simulink model "px4_mc_notch_sim"  (R2019b)
settings: Solver=FixedStepAuto  StartTime=0.0  StopTime=sim_time  FixedStep=1/sim_freq  RelTol=1e-3
values from neighbouring files (symbols this model uses):
  notch = (s^2 + wc^2)/(s^2 + o*s + wc^2)    [notch_design.m]
  pos_e_step = [0,2,0]    [run_sim.m]
  pulse_amplitude = 0.1    [run_sim.m]
  pulse_period = 40    [run_sim.m]
  ramp_max = 0.5    [run_sim.m]
  ramp_slope = 0.05    [run_sim.m]
  sinus_amplitude = 0.1    [run_sim.m]
  sinus_bias = 0    [run_sim.m]
  sinus_freq = 5    [run_sim.m]
  step_delay = 1    [run_sim.m]
  step_mag = 0.5    [run_sim.m]
  yaw_step = 0.00    (= 0)    [run_sim.m]
undefined symbols (not defined in the file or in its folder): br_filt_denom, br_filt_num, C_D, d, DiscIntNeverNeededParam, eta_w, g, hover_perc, m, max_T, MC_PITCH_P, MC_PITCHRATE_D, MC_PITCHRATE_I, MC_PITCHRATE_MAX, MC_PITCHRATE_P, MC_PR_INT_LIM, MC_ROLL_P, MC_ROLLRATE_D, MC_ROLLRATE_I, MC_ROLLRATE_MAX, MC_ROLLRATE_P, MC_RR_INT_LIM, MC_YAW_P, MC_YAWRATE_D, MC_YAWRATE_I, MC_YAWRATE_MAX, MC_YAWRATE_P, MC_YR_INT_LIM, MPC_THR_MAX, MPC_THR_MIN, MPC_TILTMAX_AIR, MPC_XY_P, MPC_XY_VEL_D, MPC_XY_VEL_I, MPC_XY_VEL_MAX, MPC_XY_VEL_P, MPC_Z_P, MPC_Z_VEL_D, MPC_Z_VEL_I, MPC_Z_VEL_MAX_DN, MPC_Z_VEL_MAX_UP, MPC_Z_VEL_P, r_D, rho, tau_T, vel_filt_denom, vel_filt_num, virtual_controls_mat, wind
libraries: simulink x7, sharedtransform x2, shared6dof x1
settings Model: Creator=henry  LastModifiedBy=henry

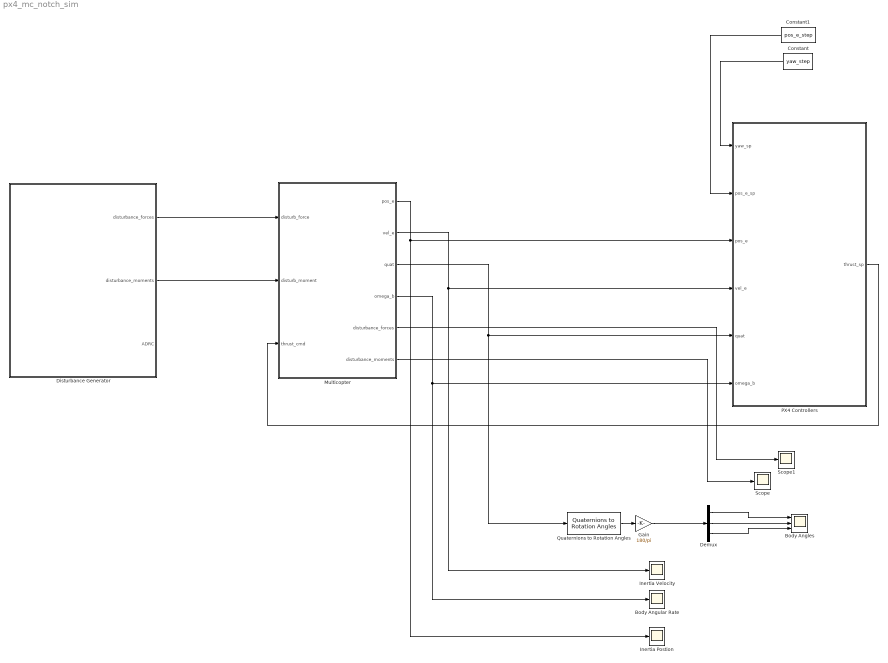
== system px4_mc_notch_sim ==
  Body Angles : Scope  NumInputPorts=3
  Body Angular Rate : Scope
  Constant : Constant  Value=yaw_step
  Constant1 : Constant  Value=pos_e_step
  Demux : Demux  Outputs=3
  Disturbance Generator : Subsystem
  Gain : Gain  Gain=180/pi
  Inertia Postion : Scope
  Inertia Velocity : Scope
  Multicopter : Subsystem
  PX4 Controllers : Subsystem
  Quaternions to Rotation Angles : sharedtransform/Quaternions to Rotation Angles  rotationOrder=XYZ  aMode=aMode
      settings: SourceProductBaseCode=AE
  Scope : Scope
  Scope1 : Scope
  wires:
  Multicopter/4(omega_b) -> Body Angular Rate/1, PX4 Controllers/6(omega_b)
  Multicopter/3("quat ") -> PX4 Controllers/5(quat), Quaternions to Rotation Angles/1
  Multicopter/1(pos_e) -> Inertia Postion/1, PX4 Controllers/3(pos_e)
  Multicopter/2(vel_e) -> PX4 Controllers/4(vel_e), Inertia Velocity/1
  PX4 Controllers/1(thrust_sp) -> Multicopter/3(thrust_cmd)
  Constant/1 -> PX4 Controllers/1(yaw_sp)
  Constant1/1 -> PX4 Controllers/2(pos_e_sp)
  Quaternions to Rotation Angles/1 -> Gain/1
  Multicopter/5(disturbance_forces) -> Scope1/1
  Gain/1 -> Demux/1
  Demux/1 -> Body Angles/1
  Demux/2 -> Body Angles/2
  Demux/3 -> Body Angles/3
  Disturbance Generator/2(disturbance_moments) -> Multicopter/2(disturb_moment)
  Disturbance Generator/1(disturbance_forces) -> Multicopter/1(disturb_force)
  Multicopter/6(disturbance_moments) -> Scope/1

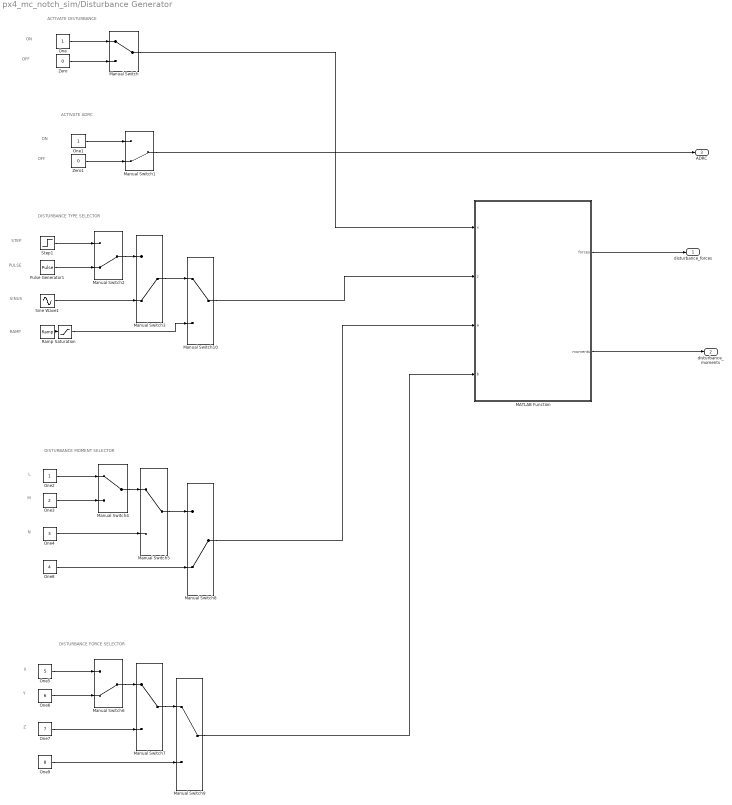
== system px4_mc_notch_sim/Disturbance Generator ==
  note: STEP
  note: OFF
  note: ON
  note: ACTIVATE DISTURBANCE
  note: DISTURBANCE TYPE SELECTOR
  note: ACTIVATE ADRC
  note: OFF
  note: ON
  note: PULSE
  note: SINUS
  note: N
  note: DISTURBANCE MOMENT SELECTOR
  note: M
  note: L
  note: Z
  note: X
  note: Y
  note: DISTURBANCE FORCE SELECTOR
  note: RAMP
  MATLAB Function : MATLAB Function  TreatAsAtomicUnit=on
  Manual Switch{,4..5,7,9..10} (6 alike) : ManualSwitch
  Manual Switch{1..3,6,8} (5 alike) : ManualSwitch  CurrentSetting=0
  One : Constant  OutDataTypeStr=Inherit: Inherit via back propagation
  One1 : Constant  OutDataTypeStr=Inherit: Inherit via back propagation
  One2 : Constant  OutDataTypeStr=Inherit: Inherit via back propagation
  One3 : Constant  Value=2  OutDataTypeStr=Inherit: Inherit via back propagation
  One4 : Constant  Value=3  OutDataTypeStr=Inherit: Inherit via back propagation
  One5 : Constant  Value=5  OutDataTypeStr=Inherit: Inherit via back propagation
  One6 : Constant  Value=6  OutDataTypeStr=Inherit: Inherit via back propagation
  One7 : Constant  Value=7  OutDataTypeStr=Inherit: Inherit via back propagation
  One8 : Constant  Value=4  OutDataTypeStr=Inherit: Inherit via back propagation
  One9 : Constant  Value=8  OutDataTypeStr=Inherit: Inherit via back propagation
  Pulse Generator1 : DiscretePulseGenerator  PulseType=Time based  Amplitude=pulse_amplitude  Period=pulse_period  PulseWidth=50
  Ramp : simulink/Sources/Ramp  slope=ramp_slope  start=ramp_start  InitialOutput=0
  Saturation : Saturate  UpperLimit=ramp_max  LowerLimit=0
  Sine Wave1 : Sin  Amplitude=sinus_amplitude  Bias=sinus_bias  Frequency=sinus_freq  SampleTime=0
  Step1 : Step  Time=step_delay  After=step_mag  SampleTime=0
  Zero : Constant  Value=0  OutDataTypeStr=Inherit: Inherit via back propagation
  Zero1 : Constant  Value=0  OutDataTypeStr=Inherit: Inherit via back propagation
  disturbance_forces : Outport
  disturbance_moments : Outport  Port=2
  ADRC : Outport  Port=3
  wires:
  One6/1 -> Manual Switch6/2
  Manual Switch7/1 -> Manual Switch9/1
  One8/1 -> Manual Switch8/2
  One7/1 -> Manual Switch7/2
  Manual Switch5/1 -> Manual Switch8/1
  One9/1 -> Manual Switch9/2
  One3/1 -> Manual Switch4/2
  Manual Switch6/1 -> Manual Switch7/1
  One5/1 -> Manual Switch6/1
  Pulse Generator1/1 -> Manual Switch2/2
  Sine Wave1/1 -> Manual Switch3/2
  Manual Switch4/1 -> Manual Switch5/1
  Manual Switch8/1 -> MATLAB Function/3(a)
  One/1 -> Manual Switch/1
  MATLAB Function/1(forces) -> disturbance_forces/1
  Zero/1 -> Manual Switch/2
  Manual Switch9/1 -> MATLAB Function/4(b)
  Zero1/1 -> Manual Switch1/2
  One4/1 -> Manual Switch5/2
  Manual Switch/1 -> MATLAB Function/1(x)
  MATLAB Function/2(moments) -> disturbance_moments/1
  Manual Switch2/1 -> Manual Switch3/1
  Step1/1 -> Manual Switch2/1
  One1/1 -> Manual Switch1/1
  One2/1 -> Manual Switch4/1
  Manual Switch1/1 -> ADRC/1
  Ramp/1 -> Saturation/1
  Manual Switch3/1 -> Manual Switch10/1
  Saturation/1 -> Manual Switch10/2
  Manual Switch10/1 -> MATLAB Function/2(z)

== system px4_mc_notch_sim/Multicopter ==
  disturb_force : Inport
  disturb_moment : Inport  Port=2
  thrust_cmd : Inport  Port=3
  6 DOF MODEL : Subsystem
  Forces and Moments : Subsystem
  Motor Model : Subsystem
  pos_e : Outport
  vel_e : Outport  Port=2
  "quat " : Outport  Port=3
  omega_b : Outport  Port=4
  disturbance_forces : Outport  Port=5
  disturbance_moments : Outport  Port=6
  wires:
  6 DOF MODEL/1(vel_b) -> Forces and Moments/1(vel_b)
  6 DOF MODEL/3(qaut) -> Forces and Moments/3(quat), "quat "/1
  6 DOF MODEL/2(pos_e) -> pos_e/1, Forces and Moments/2(pos_e)
  Forces and Moments/2(moments) -> 6 DOF MODEL/2(moments)
  6 DOF MODEL/5(omega_b) -> omega_b/1
  6 DOF MODEL/4(vel_e) -> vel_e/1
  Forces and Moments/1(forces) -> 6 DOF MODEL/1("forces ")
  thrust_cmd/1 -> Motor Model/1(thrust_cmd)
  Motor Model/1(force) -> Forces and Moments/4(thrust_cmd)
  Forces and Moments/3(disturbance_force) -> disturbance_forces/1
  Forces and Moments/4(disturbance_moments) -> disturbance_moments/1
  disturb_force/1 -> Forces and Moments/5(disturb_force)
  disturb_moment/1 -> Forces and Moments/6(disturb_moments)

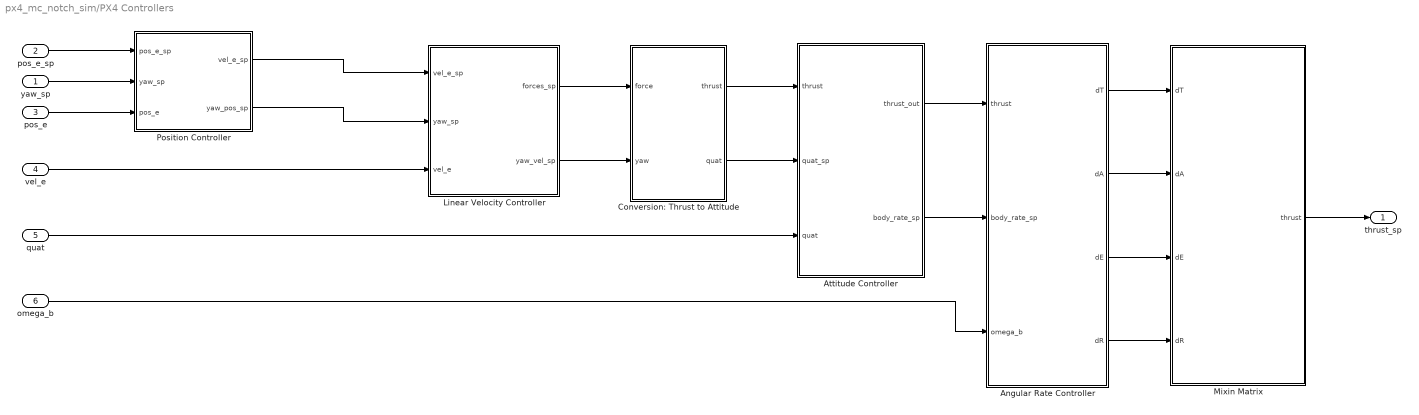
== system px4_mc_notch_sim/PX4 Controllers ==
  yaw_sp : Inport
  pos_e_sp : Inport  Port=2
  pos_e : Inport  Port=3
  vel_e : Inport  Port=4
  quat : Inport  Port=5
  omega_b : Inport  Port=6
  Angular Rate Controller : Subsystem
  Attitude Controller : Subsystem
  Conversion: Thrust to Attitude : Subsystem
  Linear Velocity Controller : Subsystem
  Mixin Matrix : Subsystem
  Position Controller : Subsystem
  thrust_sp : Outport
  wires:
  yaw_sp/1 -> Position Controller/2(yaw_sp)
  pos_e_sp/1 -> Position Controller/1(pos_e_sp)
  quat/1 -> Attitude Controller/3(quat)
  omega_b/1 -> Angular Rate Controller/3(omega_b)
  pos_e/1 -> Position Controller/3(pos_e)
  vel_e/1 -> Linear Velocity Controller/3(vel_e)
  Position Controller/2(yaw_pos_sp) -> Linear Velocity Controller/2(yaw_sp)
  Position Controller/1(vel_e_sp) -> Linear Velocity Controller/1(vel_e_sp)
  Linear Velocity Controller/1(forces_sp) -> Conversion: Thrust to Attitude/1(force)
  Linear Velocity Controller/2(yaw_vel_sp) -> Conversion: Thrust to Attitude/2(yaw)
  Conversion: Thrust to Attitude/1(thrust) -> Attitude Controller/1(thrust)
  Conversion: Thrust to Attitude/2(quat) -> Attitude Controller/2(quat_sp)
  Attitude Controller/1(thrust_out) -> Angular Rate Controller/1(thrust)
  Attitude Controller/2(body_rate_sp) -> Angular Rate Controller/2(body_rate_sp)
  Angular Rate Controller/1(dT) -> Mixin Matrix/1(dT)
  Angular Rate Controller/2(dA) -> Mixin Matrix/2(dA)
  Angular Rate Controller/3(dE) -> Mixin Matrix/3(dE)
  Angular Rate Controller/4(dR) -> Mixin Matrix/4(dR)
  Mixin Matrix/1(thrust) -> thrust_sp/1

== system px4_mc_notch_sim/Multicopter/6 DOF MODEL ==
  "forces " : Inport
  moments : Inport  Port=2
  6DOF (Quaternion) : shared6dof/6DOF (Euler Angles)  units=Metric (MKS)  mtype=Fixed  rep=Quaternion  xme_0=[0 0 0]  Vm_0=[0 0 0]  eul_0=[0 0 0]  pm_0=[0 0 0]  mass_0=m  mass_e=0.5  mass_f=2.0  inertia=I  inertia_e=eye(3)  inertia_f=2*eye(3)  k_quat=2  vre_flag=on  abi_flag=off  aMode=0  xme_statename=''  Vm_statename=''  eul_statename=''  quat_statename=''  pm_statename=''  mass_statename=''
      settings: SourceProductBaseCode=AE
  Direction Cosine Matrix to Quaternions : sharedtransform/Direction Cosine Matrix  to Quaternions  aMode=0  action=None  tolerance=eps(2)
      settings: SourceProductName=Aerospace Blockset  SourceProductBaseCode=AE
  Terminator : Terminator
  Terminator1 : Terminator
  Terminator2 : Terminator
  vel_b : Outport
  pos_e : Outport  Port=2
  qaut : Outport  Port=3
  vel_e : Outport  Port=4
  omega_b : Outport  Port=5
  wires:
  "forces "/1 -> 6DOF (Quaternion)/1
  moments/1 -> 6DOF (Quaternion)/2
  6DOF (Quaternion)/8 -> Terminator/1
  6DOF (Quaternion)/7 -> Terminator1/1
  6DOF (Quaternion)/3 -> Terminator2/1
  6DOF (Quaternion)/1 -> vel_e/1
  6DOF (Quaternion)/2 -> pos_e/1
  6DOF (Quaternion)/5 -> vel_b/1
  6DOF (Quaternion)/6 -> omega_b/1
  Direction Cosine Matrix to Quaternions/1 -> qaut/1
  6DOF (Quaternion)/4 -> Direction Cosine Matrix to Quaternions/1

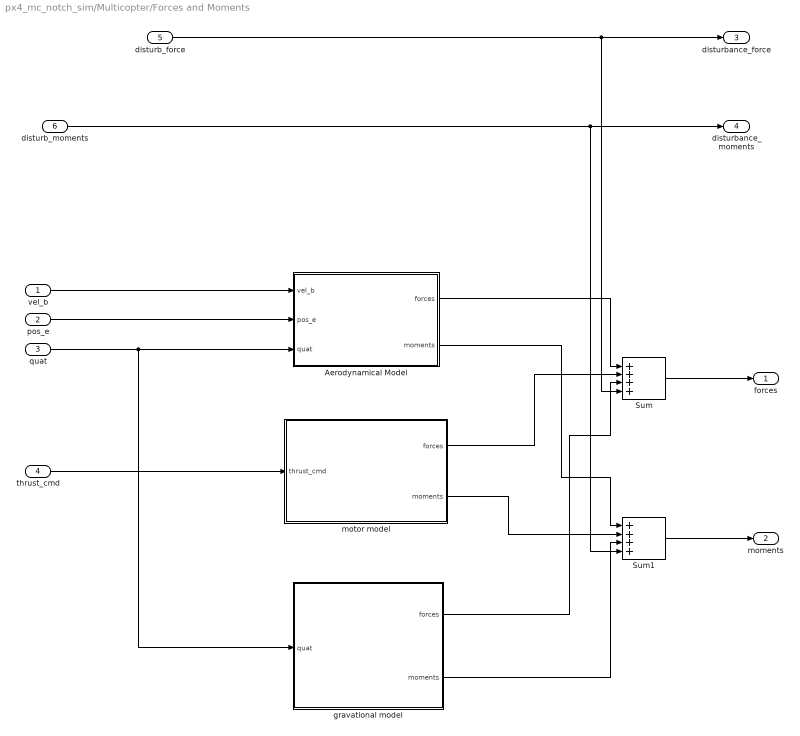
== system px4_mc_notch_sim/Multicopter/Forces and Moments ==
  vel_b : Inport
  pos_e : Inport  Port=2
  quat : Inport  Port=3
  thrust_cmd : Inport  Port=4
  disturb_force : Inport  Port=5
  disturb_moments : Inport  Port=6
  Aerodynamical Model : Subsystem
  Sum : Sum  Inputs=++++
  Sum1 : Sum  Inputs=++++
  gravational model : Subsystem
  motor model : Subsystem
  forces : Outport
  moments : Outport  Port=2
  disturbance_force : Outport  Port=3
  disturbance_moments : Outport  Port=4
  wires:
  Sum/1 -> forces/1
  Sum1/1 -> moments/1
  motor model/1(forces) -> Sum/2
  motor model/2(moments) -> Sum1/2
  gravational model/1(forces) -> Sum/3
  gravational model/2(moments) -> Sum1/3
  vel_b/1 -> Aerodynamical Model/1(vel_b)
  pos_e/1 -> Aerodynamical Model/2(pos_e)
  Aerodynamical Model/1(forces) -> Sum/1
  Aerodynamical Model/2(moments) -> Sum1/1
  thrust_cmd/1 -> motor model/1(thrust_cmd)
  disturb_moments/1 -> Sum1/4, disturbance_moments/1
  quat/1 -> Aerodynamical Model/3(quat), gravational model/1(quat)
  disturb_force/1 -> Sum/4, disturbance_force/1

== system px4_mc_notch_sim/Multicopter/Motor Model ==
  thrust_cmd : Inport
  Linear Gain : Gain  Gain=max_T
  force : Outport  VectorParamsAs1DForOutWhenUnconnected=off
  wires:
  thrust_cmd/1 -> Linear Gain/1
  Linear Gain/1 -> force/1

== system px4_mc_notch_sim/PX4 Controllers/Angular Rate Controller ==
  thrust : Inport
  body_rate_sp : Inport  Port=2
  omega_b : Inport  Port=3
  Demux : Demux  Outputs=3
  Demux1 : Demux  Outputs=3
  Pitch Rate Controller : Subsystem
  Roll Rate Controller : Subsystem
  Yaw Rate Controller : Subsystem
  dT : Outport  VectorParamsAs1DForOutWhenUnconnected=off
  dA : Outport  Port=2  VectorParamsAs1DForOutWhenUnconnected=off
  dE : Outport  Port=3  VectorParamsAs1DForOutWhenUnconnected=off
  dR : Outport  Port=4  VectorParamsAs1DForOutWhenUnconnected=off
  wires:
  Demux1/3 -> Yaw Rate Controller/2(r)
  Demux/3 -> Yaw Rate Controller/1(rref)
  Demux1/1 -> Roll Rate Controller/2(p)
  thrust/1 -> dT/1
  Yaw Rate Controller/1(dR) -> dR/1
  Pitch Rate Controller/1(dE) -> dE/1
  Demux1/2 -> Pitch Rate Controller/2(q)
  Roll Rate Controller/1(dA) -> dA/1
  Demux/1 -> Roll Rate Controller/1(pref)
  Demux/2 -> Pitch Rate Controller/1(qref)
  omega_b/1 -> Demux1/1
  body_rate_sp/1 -> Demux/1

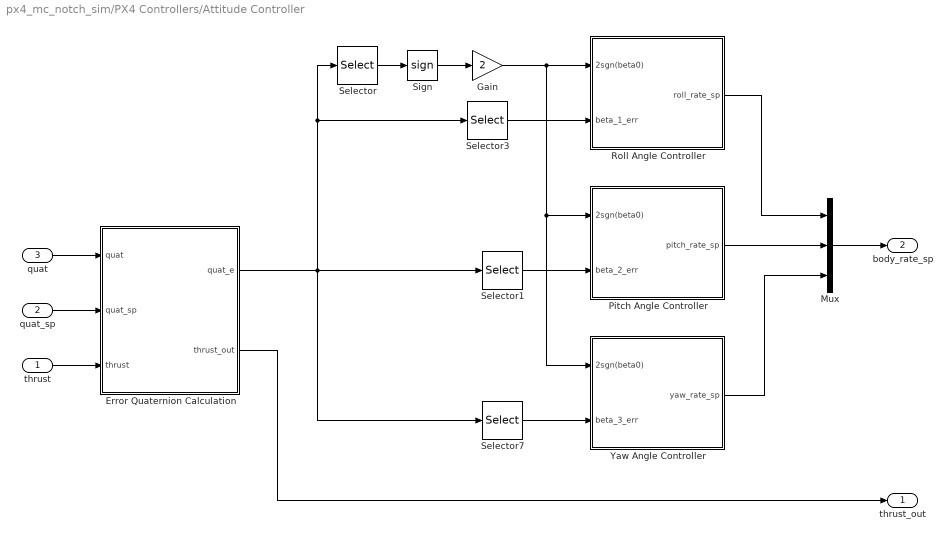
== system px4_mc_notch_sim/PX4 Controllers/Attitude Controller ==
  thrust : Inport  PortDimensions=1
  quat_sp : Inport  Port=2  PortDimensions=4
  quat : Inport  Port=3  PortDimensions=4
  Error Quaternion Calculation : MATLAB Function  TreatAsAtomicUnit=on
  Gain : Gain  Gain=2
  Mux : Mux  Inputs=3
  Pitch Angle Controller : Subsystem
  Roll Angle Controller : Subsystem
  Selector : Selector  InputPortWidth=4  IndexOptions=Index vector (dialog)  Indices=1  OutputSizes=1
  Selector1 : Selector  InputPortWidth=4  IndexOptions=Index vector (dialog)  Indices=3  OutputSizes=1
  Selector3 : Selector  InputPortWidth=4  IndexOptions=Index vector (dialog)  Indices=2  OutputSizes=1
  Selector7 : Selector  InputPortWidth=4  IndexOptions=Index vector (dialog)  Indices=4  OutputSizes=1
  Sign : Signum
  Yaw Angle Controller : Subsystem
  thrust_out : Outport  VectorParamsAs1DForOutWhenUnconnected=off
  body_rate_sp : Outport  Port=2  VectorParamsAs1DForOutWhenUnconnected=off
  wires:
  Pitch Angle Controller/1(pitch_rate_sp) -> Mux/2
  Selector7/1 -> Yaw Angle Controller/2(beta_3_err)
  Mux/1 -> body_rate_sp/1
  quat/1 -> Error Quaternion Calculation/1(quat)
  quat_sp/1 -> Error Quaternion Calculation/2(quat_sp)
  Error Quaternion Calculation/1(quat_e) -> Selector7/1, Selector/1, Selector3/1, Selector1/1
  Selector/1 -> Sign/1
  Yaw Angle Controller/1(yaw_rate_sp) -> Mux/3
  Roll Angle Controller/1(roll_rate_sp) -> Mux/1
  Selector3/1 -> Roll Angle Controller/2(beta_1_err)
  Gain/1 -> Yaw Angle Controller/1(2sgn(beta0)), Pitch Angle Controller/1(2sgn(beta0)), Roll Angle Controller/1(2sgn(beta0))
  thrust/1 -> Error Quaternion Calculation/3(thrust)
  Sign/1 -> Gain/1
  Error Quaternion Calculation/2(thrust_out) -> thrust_out/1
  Selector1/1 -> Pitch Angle Controller/2(beta_2_err)

== system px4_mc_notch_sim/PX4 Controllers/Conversion: Thrust to Attitude ==
  force : Inport
  yaw : Inport  Port=2
  thrust2att : MATLAB Function  TreatAsAtomicUnit=on
  thrust : Outport  VectorParamsAs1DForOutWhenUnconnected=off
  quat : Outport  Port=2  VectorParamsAs1DForOutWhenUnconnected=off
  wires:
  yaw/1 -> thrust2att/2(yaw)
  force/1 -> thrust2att/1(force)
  thrust2att/2(thrust) -> thrust/1
  thrust2att/1(quat) -> quat/1

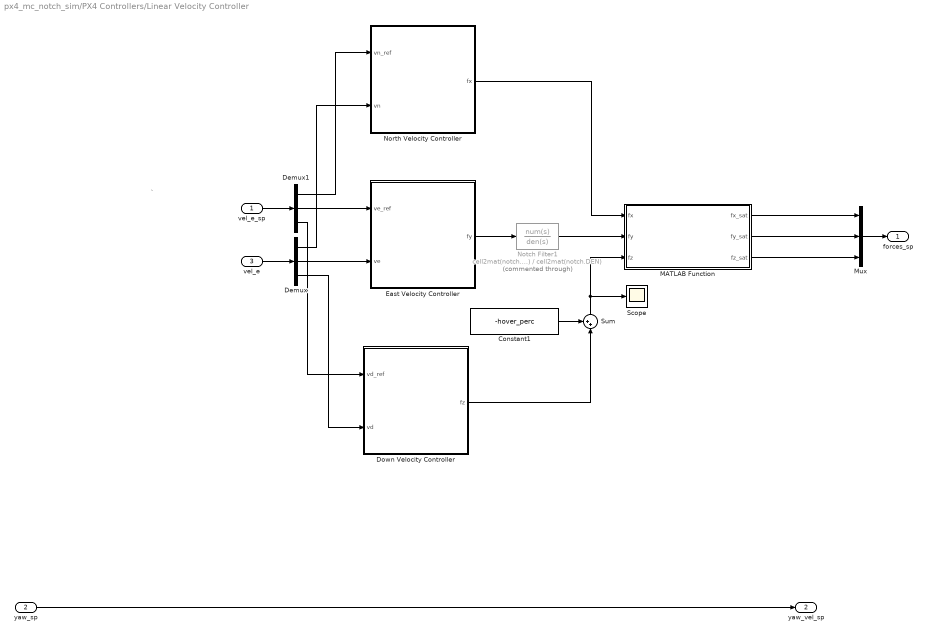
== system px4_mc_notch_sim/PX4 Controllers/Linear Velocity Controller ==
  note: `
  vel_e_sp : Inport
  yaw_sp : Inport  Port=2
  vel_e : Inport  Port=3
  Constant1 : Constant  Value=-hover_perc
  Demux : Demux  Outputs=3
  Demux1 : Demux  Outputs=3
  Down Velocity Controller : Subsystem
  East Velocity Controller : Subsystem
  MATLAB Function : MATLAB Function  TreatAsAtomicUnit=on
  Mux : Mux  Inputs=3
  North Velocity Controller : Subsystem
  Notch Filter1 : TransferFcn  Commented=through  Numerator=cell2mat(notch.NUM)  Denominator=cell2mat(notch.DEN)
  Scope : Scope
  Sum : Sum  Inputs=++|
  forces_sp : Outport  VectorParamsAs1DForOutWhenUnconnected=off
  yaw_vel_sp : Outport  Port=2  VectorParamsAs1DForOutWhenUnconnected=off
  wires:
  Mux/1 -> forces_sp/1
  Demux/2 -> East Velocity Controller/2(ve)
  vel_e_sp/1 -> Demux1/1
  Down Velocity Controller/1(fz) -> Sum/2
  Demux1/1 -> North Velocity Controller/1(vn_ref)
  Constant1/1 -> Sum/1
  Demux/1 -> North Velocity Controller/2(vn)
  Demux/3 -> Down Velocity Controller/2(vd)
  vel_e/1 -> Demux/1
  East Velocity Controller/1(fy) -> Notch Filter1/1
  yaw_sp/1 -> yaw_vel_sp/1
  Demux1/3 -> Down Velocity Controller/1(vd_ref)
  Demux1/2 -> East Velocity Controller/1(ve_ref)
  MATLAB Function/3(fz_sat) -> Mux/3
  Sum/1 -> Scope/1, MATLAB Function/3(fz)
  MATLAB Function/2(fy_sat) -> Mux/2
  MATLAB Function/1(fx_sat) -> Mux/1
  North Velocity Controller/1(fx) -> MATLAB Function/1(fx)
  Notch Filter1/1 -> MATLAB Function/2(fy)

== system px4_mc_notch_sim/PX4 Controllers/Mixin Matrix ==
  dT : Inport
  dA : Inport  Port=2
  dE : Inport  Port=3
  dR : Inport  Port=4
  Mixin_mat : MATLAB Function  TreatAsAtomicUnit=on
  Precision Conversion : Subsystem
  Saturation : Saturate  UpperLimit=1  LowerLimit=0
  thrust : Outport  VectorParamsAs1DForOutWhenUnconnected=off
  wires:
  Mixin_mat/1(thrust) -> Saturation/1
  dT/1 -> Mixin_mat/1(dT)
  Saturation/1 -> Precision Conversion/1(analog_cmd)
  dE/1 -> Mixin_mat/3(dE)
  dA/1 -> Mixin_mat/2(dA)
  dR/1 -> Mixin_mat/4(dR)
  Precision Conversion/1(discrete_cmd) -> thrust/1

== system px4_mc_notch_sim/PX4 Controllers/Position Controller ==
  pos_e_sp : Inport
  yaw_sp : Inport  Port=2
  pos_e : Inport  Port=3
  Demux : Demux  Outputs=3
  Demux1 : Demux  Outputs=3
  Down Position Controller : Subsystem
  East Position Controller : Subsystem
  Mux : Mux  Inputs=3
  North Position Controller : Subsystem
  Notch Filter1 : TransferFcn  Numerator=cell2mat(notch.NUM)  Denominator=cell2mat(notch.DEN)
  vel_e_sp : Outport  VectorParamsAs1DForOutWhenUnconnected=off
  yaw_pos_sp : Outport  Port=2  VectorParamsAs1DForOutWhenUnconnected=off
  wires:
  Demux/1 -> North Position Controller/1(n_ref)
  North Position Controller/1(vn) -> Mux/1
  pos_e_sp/1 -> Demux/1
  yaw_sp/1 -> yaw_pos_sp/1
  Demux1/1 -> North Position Controller/2(n)
  Demux/2 -> East Position Controller/1(e_ref)
  Down Position Controller/1(vd) -> Mux/3
  Demux1/2 -> East Position Controller/2(e)
  Demux/3 -> Down Position Controller/1(d_ref)
  Mux/1 -> vel_e_sp/1
  East Position Controller/1(ve) -> Notch Filter1/1
  Demux1/3 -> Down Position Controller/2(d)
  pos_e/1 -> Demux1/1
  Notch Filter1/1 -> Mux/2

== system px4_mc_notch_sim/Multicopter/Forces and Moments/Aerodynamical Model ==
  vel_b : Inport
  pos_e : Inport  Port=2
  quat : Inport  Port=3
  Constant : Constant  Value=wind
  aerodynamic_model : MATLAB Function  TreatAsAtomicUnit=on
  forces : Outport
  moments : Outport  Port=2
  wires:
  quat/1 -> aerodynamic_model/4(quat)
  aerodynamic_model/2(moments) -> moments/1
  vel_b/1 -> aerodynamic_model/1(v_b)
  aerodynamic_model/1(forces) -> forces/1
  pos_e/1 -> aerodynamic_model/3(ned)
  Constant/1 -> aerodynamic_model/2(vw_i)

== system px4_mc_notch_sim/Multicopter/Forces and Moments/gravational model ==
  quat : Inport
  gravitional_model : MATLAB Function  TreatAsAtomicUnit=on
  forces : Outport
  moments : Outport  Port=2
  wires:
  gravitional_model/1(forces) -> forces/1
  gravitional_model/2(moments) -> moments/1
  quat/1 -> gravitional_model/1(quat)

== system px4_mc_notch_sim/Multicopter/Forces and Moments/motor model ==
  thrust_cmd : Inport
  Integrator : Integrator
  thrust_model : MATLAB Function  TreatAsAtomicUnit=on
  forces : Outport
  moments : Outport  Port=2
  wires:
  thrust_model/3(moments) -> moments/1
  thrust_cmd/1 -> thrust_model/2(T_cmd)
  Integrator/1 -> thrust_model/1(T)
  thrust_model/2(forces) -> forces/1
  thrust_model/1(T_dot) -> Integrator/1

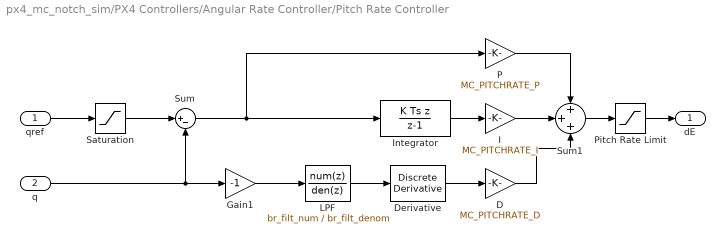
== system px4_mc_notch_sim/PX4 Controllers/Angular Rate Controller/Pitch Rate Controller ==
  qref : Inport
  q : Inport  Port=2
  D : Gain  Gain=MC_PITCHRATE_D
  Derivative : simulink/Discrete/Discrete Derivative  gainval=1  ICPrevScaledInput=0.0  OutMin=[]  OutMax=[]  OutDataType=fixdt(1, 16)  OutScaling=2^-10  DoSatur=off
  Gain1 : Gain  Gain=-1
  I : Gain  Gain=MC_PITCHRATE_I
  Integrator : DiscreteIntegrator  IntegratorMethod=Integration: Backward Euler  gainval=1  SampleTime=-1  LimitOutput=on  UpperSaturationLimit=MC_PR_INT_LIM  LowerSaturationLimit=-MC_PR_INT_LIM  ICPrevOutput=DiscIntNeverNeededParam  ICPrevScaledInput=DiscIntNeverNeededParam
  LPF : DiscreteTransferFcn  Numerator=br_filt_num  Denominator=br_filt_denom
  P : Gain  Gain=MC_PITCHRATE_P
  Pitch Rate Limit : Saturate  UpperLimit=1  LowerLimit=-1
  Saturation : Saturate  UpperLimit=MC_PITCHRATE_MAX*pi/180  LowerLimit=-MC_PITCHRATE_MAX*pi/180
  Sum : Sum  Inputs=|+-
  Sum1 : Sum  Inputs=+++
  dE : Outport  VectorParamsAs1DForOutWhenUnconnected=off
  wires:
  Gain1/1 -> LPF/1
  P/1 -> Sum1/1
  Sum1/1 -> Pitch Rate Limit/1
  Saturation/1 -> Sum/1
  I/1 -> Sum1/2
  Sum/1 -> Integrator/1, P/1
  Derivative/1 -> D/1
  D/1 -> Sum1/3
  qref/1 -> Saturation/1
  q/1 -> Gain1/1, Sum/2
  LPF/1 -> Derivative/1
  Integrator/1 -> I/1
  Pitch Rate Limit/1 -> dE/1

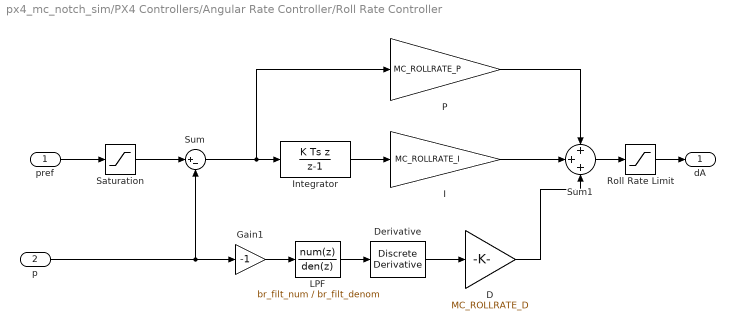
== system px4_mc_notch_sim/PX4 Controllers/Angular Rate Controller/Roll Rate Controller ==
  pref : Inport
  p : Inport  Port=2
  D : Gain  Gain=MC_ROLLRATE_D
  Derivative : simulink/Discrete/Discrete Derivative  gainval=1  ICPrevScaledInput=0.0  OutMin=[]  OutMax=[]  OutDataType=fixdt(1, 16)  OutScaling=2^-10  DoSatur=off
  Gain1 : Gain  Gain=-1
  I : Gain  Gain=MC_ROLLRATE_I
  Integrator : DiscreteIntegrator  IntegratorMethod=Integration: Backward Euler  gainval=1  SampleTime=-1  LimitOutput=on  UpperSaturationLimit=MC_RR_INT_LIM  LowerSaturationLimit=-MC_RR_INT_LIM  ICPrevOutput=DiscIntNeverNeededParam  ICPrevScaledInput=DiscIntNeverNeededParam
  LPF : DiscreteTransferFcn  Numerator=br_filt_num  Denominator=br_filt_denom
  P : Gain  Gain=MC_ROLLRATE_P
  Roll Rate Limit : Saturate  UpperLimit=1  LowerLimit=-1
  Saturation : Saturate  UpperLimit=MC_ROLLRATE_MAX*pi/180  LowerLimit=-MC_ROLLRATE_MAX*pi/180
  Sum : Sum  Inputs=|+-
  Sum1 : Sum  Inputs=+++
  dA : Outport  VectorParamsAs1DForOutWhenUnconnected=off
  wires:
  Gain1/1 -> LPF/1
  P/1 -> Sum1/1
  Sum1/1 -> Roll Rate Limit/1
  Saturation/1 -> Sum/1
  I/1 -> Sum1/2
  Sum/1 -> P/1, Integrator/1
  Derivative/1 -> D/1
  D/1 -> Sum1/3
  pref/1 -> Saturation/1
  p/1 -> Gain1/1, Sum/2
  LPF/1 -> Derivative/1
  Integrator/1 -> I/1
  Roll Rate Limit/1 -> dA/1

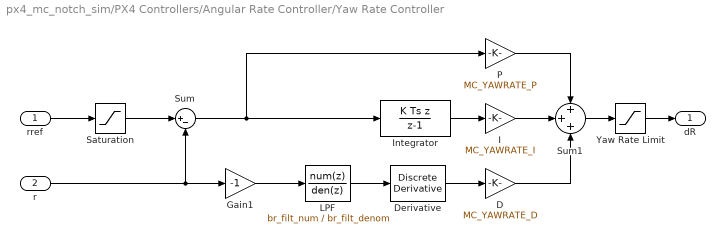
== system px4_mc_notch_sim/PX4 Controllers/Angular Rate Controller/Yaw Rate Controller ==
  rref : Inport
  r : Inport  Port=2
  D : Gain  Gain=MC_YAWRATE_D
  Derivative : simulink/Discrete/Discrete Derivative  gainval=1  ICPrevScaledInput=0.0  OutMin=[]  OutMax=[]  OutDataType=fixdt(1, 16)  OutScaling=2^-10  DoSatur=off
  Gain1 : Gain  Gain=-1
  I : Gain  Gain=MC_YAWRATE_I
  Integrator : DiscreteIntegrator  IntegratorMethod=Integration: Backward Euler  gainval=1  SampleTime=-1  LimitOutput=on  UpperSaturationLimit=MC_YR_INT_LIM  LowerSaturationLimit=-MC_YR_INT_LIM  ICPrevOutput=DiscIntNeverNeededParam  ICPrevScaledInput=DiscIntNeverNeededParam
  LPF : DiscreteTransferFcn  Numerator=br_filt_num  Denominator=br_filt_denom
  P : Gain  Gain=MC_YAWRATE_P
  Saturation : Saturate  UpperLimit=MC_YAWRATE_MAX*pi/180  LowerLimit=-MC_YAWRATE_MAX*pi/180
  Sum : Sum  Inputs=|+-
  Sum1 : Sum  Inputs=+++
  Yaw Rate Limit : Saturate  UpperLimit=1  LowerLimit=-1
  dR : Outport  VectorParamsAs1DForOutWhenUnconnected=off
  wires:
  Gain1/1 -> LPF/1
  P/1 -> Sum1/1
  Sum1/1 -> Yaw Rate Limit/1
  Saturation/1 -> Sum/1
  I/1 -> Sum1/2
  Sum/1 -> Integrator/1, P/1
  Derivative/1 -> D/1
  D/1 -> Sum1/3
  rref/1 -> Saturation/1
  r/1 -> Gain1/1, Sum/2
  LPF/1 -> Derivative/1
  Integrator/1 -> I/1
  Yaw Rate Limit/1 -> dR/1

== system px4_mc_notch_sim/PX4 Controllers/Attitude Controller/Pitch Angle Controller ==
  2sgn(beta0) : Inport
  beta_2_err : Inport  Port=2
  Multiply : Product
  P : Gain  Gain=MC_PITCH_P
  pitch_rate_sp : Outport  VectorParamsAs1DForOutWhenUnconnected=off
  wires:
  P/1 -> Multiply/1
  beta_2_err/1 -> P/1
  2sgn(beta0)/1 -> Multiply/2
  Multiply/1 -> pitch_rate_sp/1

== system px4_mc_notch_sim/PX4 Controllers/Attitude Controller/Roll Angle Controller ==
  2sgn(beta0) : Inport
  beta_1_err : Inport  Port=2
  Multiply : Product
  P : Gain  Gain=MC_ROLL_P
  roll_rate_sp : Outport  VectorParamsAs1DForOutWhenUnconnected=off
  wires:
  P/1 -> Multiply/1
  beta_1_err/1 -> P/1
  2sgn(beta0)/1 -> Multiply/2
  Multiply/1 -> roll_rate_sp/1

== system px4_mc_notch_sim/PX4 Controllers/Attitude Controller/Yaw Angle Controller ==
  2sgn(beta0) : Inport
  beta_3_err : Inport  Port=2
  Multiply : Product
  P : Gain  Gain=MC_YAW_P
  yaw_rate_sp : Outport  VectorParamsAs1DForOutWhenUnconnected=off
  wires:
  P/1 -> Multiply/1
  beta_3_err/1 -> P/1
  2sgn(beta0)/1 -> Multiply/2
  Multiply/1 -> yaw_rate_sp/1

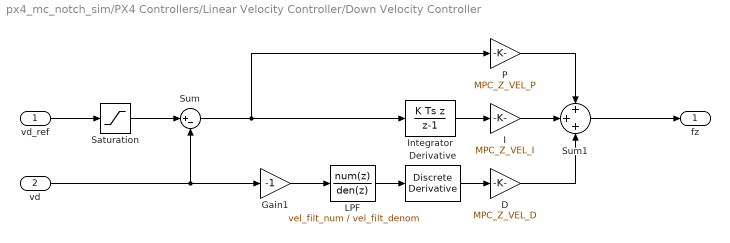
== system px4_mc_notch_sim/PX4 Controllers/Linear Velocity Controller/Down Velocity Controller ==
  vd_ref : Inport
  vd : Inport  Port=2
  D : Gain  Gain=MPC_Z_VEL_D
  Derivative : simulink/Discrete/Discrete Derivative  gainval=1  ICPrevScaledInput=0.0  OutMin=[]  OutMax=[]  OutDataType=fixdt(1, 16)  OutScaling=2^-10  DoSatur=off
  Gain1 : Gain  Gain=-1
  I : Gain  Gain=MPC_Z_VEL_I
  Integrator : DiscreteIntegrator  IntegratorMethod=Integration: Backward Euler  gainval=1  SampleTime=-1  UpperSaturationLimit=MC_PR_INT_LIM  LowerSaturationLimit=-MC_PR_INT_LIM  ICPrevOutput=DiscIntNeverNeededParam  ICPrevScaledInput=DiscIntNeverNeededParam
  LPF : DiscreteTransferFcn  Numerator=vel_filt_num  Denominator=vel_filt_denom
  P : Gain  Gain=MPC_Z_VEL_P
  Saturation : Saturate  UpperLimit=MPC_Z_VEL_MAX_UP  LowerLimit=-MPC_Z_VEL_MAX_DN
  Sum : Sum  Inputs=|+-
  Sum1 : Sum  Inputs=+++
  fz : Outport  VectorParamsAs1DForOutWhenUnconnected=off
  wires:
  vd_ref/1 -> Saturation/1
  P/1 -> Sum1/1
  Sum1/1 -> fz/1
  vd/1 -> Sum/2, Gain1/1
  Gain1/1 -> LPF/1
  LPF/1 -> Derivative/1
  D/1 -> Sum1/3
  Saturation/1 -> Sum/1
  I/1 -> Sum1/2
  Integrator/1 -> I/1
  Sum/1 -> Integrator/1, P/1
  Derivative/1 -> D/1

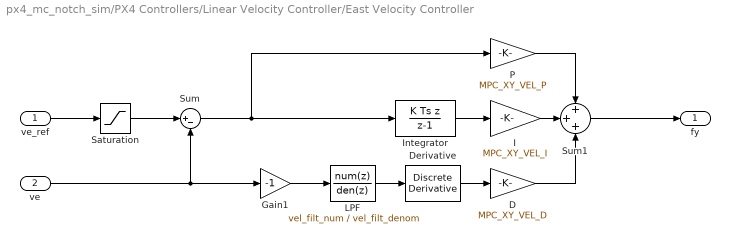
== system px4_mc_notch_sim/PX4 Controllers/Linear Velocity Controller/East Velocity Controller ==
  ve_ref : Inport
  ve : Inport  Port=2
  D : Gain  Gain=MPC_XY_VEL_D
  Derivative : simulink/Discrete/Discrete Derivative  gainval=1  ICPrevScaledInput=0.0  OutMin=[]  OutMax=[]  OutDataType=fixdt(1, 16)  OutScaling=2^-10  DoSatur=off
  Gain1 : Gain  Gain=-1
  I : Gain  Gain=MPC_XY_VEL_I
  Integrator : DiscreteIntegrator  IntegratorMethod=Integration: Backward Euler  gainval=1  SampleTime=-1  UpperSaturationLimit=MC_PR_INT_LIM  LowerSaturationLimit=-MC_PR_INT_LIM  ICPrevOutput=DiscIntNeverNeededParam  ICPrevScaledInput=DiscIntNeverNeededParam
  LPF : DiscreteTransferFcn  Numerator=vel_filt_num  Denominator=vel_filt_denom
  P : Gain  Gain=MPC_XY_VEL_P
  Saturation : Saturate  UpperLimit=MPC_XY_VEL_MAX  LowerLimit=-MPC_XY_VEL_MAX
  Sum : Sum  Inputs=|+-
  Sum1 : Sum  Inputs=+++
  fy : Outport  VectorParamsAs1DForOutWhenUnconnected=off
  wires:
  ve_ref/1 -> Saturation/1
  P/1 -> Sum1/1
  Sum1/1 -> fy/1
  ve/1 -> Sum/2, Gain1/1
  Gain1/1 -> LPF/1
  LPF/1 -> Derivative/1
  D/1 -> Sum1/3
  Saturation/1 -> Sum/1
  I/1 -> Sum1/2
  Integrator/1 -> I/1
  Sum/1 -> Integrator/1, P/1
  Derivative/1 -> D/1

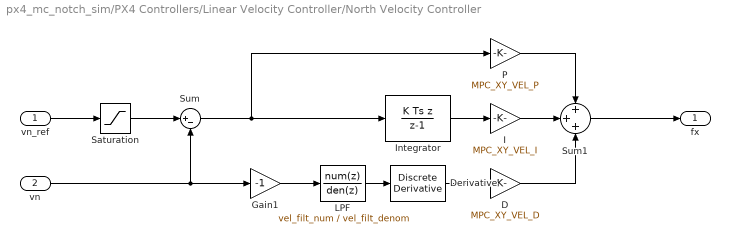
== system px4_mc_notch_sim/PX4 Controllers/Linear Velocity Controller/North Velocity Controller ==
  vn_ref : Inport
  vn : Inport  Port=2
  D : Gain  Gain=MPC_XY_VEL_D
  Derivative : simulink/Discrete/Discrete Derivative  gainval=1  ICPrevScaledInput=0.0  OutMin=[]  OutMax=[]  OutDataType=fixdt(1, 16)  OutScaling=2^-10  DoSatur=off
  Gain1 : Gain  Gain=-1
  I : Gain  Gain=MPC_XY_VEL_I
  Integrator : DiscreteIntegrator  IntegratorMethod=Integration: Backward Euler  gainval=1  SampleTime=-1  UpperSaturationLimit=MC_PR_INT_LIM  LowerSaturationLimit=-MC_PR_INT_LIM  ICPrevOutput=DiscIntNeverNeededParam  ICPrevScaledInput=DiscIntNeverNeededParam
  LPF : DiscreteTransferFcn  Numerator=vel_filt_num  Denominator=vel_filt_denom
  P : Gain  Gain=MPC_XY_VEL_P
  Saturation : Saturate  UpperLimit=MPC_XY_VEL_MAX  LowerLimit=-MPC_XY_VEL_MAX
  Sum : Sum  Inputs=|+-
  Sum1 : Sum  Inputs=+++
  fx : Outport  VectorParamsAs1DForOutWhenUnconnected=off
  wires:
  vn_ref/1 -> Saturation/1
  P/1 -> Sum1/1
  Sum1/1 -> fx/1
  vn/1 -> Sum/2, Gain1/1
  LPF/1 -> Derivative/1
  D/1 -> Sum1/3
  Saturation/1 -> Sum/1
  I/1 -> Sum1/2
  Integrator/1 -> I/1
  Sum/1 -> Integrator/1, P/1
  Derivative/1 -> D/1
  Gain1/1 -> LPF/1

== system px4_mc_notch_sim/PX4 Controllers/Mixin Matrix/Precision Conversion ==
  analog_cmd : Inport
  Gain : Gain  Gain=10000
  Gain1 : Gain  Gain=1/10000
  Round : Rounding
  discrete_cmd : Outport  VectorParamsAs1DForOutWhenUnconnected=off
  wires:
  analog_cmd/1 -> Gain/1
  Gain/1 -> Round/1
  Round/1 -> Gain1/1
  Gain1/1 -> discrete_cmd/1

== system px4_mc_notch_sim/PX4 Controllers/Position Controller/Down Position Controller ==
  d_ref : Inport
  d : Inport  Port=2
  P : Gain  Gain=MPC_Z_P
  Sum : Sum  Inputs=|+-
  vd : Outport  VectorParamsAs1DForOutWhenUnconnected=off
  wires:
  d/1 -> Sum/2
  d_ref/1 -> Sum/1
  Sum/1 -> P/1
  P/1 -> vd/1

== system px4_mc_notch_sim/PX4 Controllers/Position Controller/East Position Controller ==
  e_ref : Inport
  e : Inport  Port=2
  P : Gain  Gain=MPC_XY_P
  Sum : Sum  Inputs=|+-
  ve : Outport  VectorParamsAs1DForOutWhenUnconnected=off
  wires:
  e/1 -> Sum/2
  e_ref/1 -> Sum/1
  Sum/1 -> P/1
  P/1 -> ve/1

== system px4_mc_notch_sim/PX4 Controllers/Position Controller/North Position Controller ==
  n_ref : Inport
  n : Inport  Port=2
  P : Gain  Gain=MPC_XY_P
  Sum : Sum  Inputs=|+-
  vn : Outport  VectorParamsAs1DForOutWhenUnconnected=off
  wires:
  n/1 -> Sum/2
  n_ref/1 -> Sum/1
  Sum/1 -> P/1
  P/1 -> vn/1

== matlab function px4_mc_notch_sim/Multicopter/Forces and Moments/motor model/thrust_model ==
  data: T input; T_cmd input; T_dot output; forces output; moments output; virtual_controls_mat parameter; tau_T parameter; d parameter; r_D parameter
function [T_dot, forces, moments] = thrust_model(T, T_cmd,virtual_controls_mat,tau_T, d,r_D)

    virt_T = virtual_controls_mat * T;

    T_dot = (-T + T_cmd)/tau_T;
    forces = [0; 0; -virt_T(1)];
    moments = [d*virt_T(2); d*virt_T(3); r_D*virt_T(4)];
    
end

== matlab function px4_mc_notch_sim/Multicopter/Forces and Moments/Aerodynamical Model/aerodynamic_model ==
  data: v_b input; forces output; vw_i input; ned input; quat input; moments output; rho parameter; C_D parameter; eta_w parameter
function [forces,moments] = aerodynamic_model(v_b, vw_i, ned, quat, rho, C_D, eta_w)
    coder.extrinsic("quatrotate");
    
    % Initialize
    vw_b = [0; 0; 0];
    
    vw_b = quatrotate(quat', vw_i')';
    vw_bm = (power(abs(ned(3))/10, eta_w)) .* vw_b;
    v_bw = -v_b + vw_bm;
    q = 0.5 * rho * v_bw.*abs(v_bw);
    
    forces = q.*C_D;
    moments = [0; 0; 0];
    
end

== matlab function px4_mc_notch_sim/Multicopter/Forces and Moments/gravational model/gravitional_model ==
  data: quat input; forces output; moments output; g parameter; m parameter
function [forces,moments] = gravitional_model(quat, g, m)
    coder.extrinsic("quatrotate");

    % Initialize
    forces = [0; 0; 0];
    
    moments = [0 ; 0 ; 0];
    forces = quatrotate(quat', [0 ; 0 ; m*g]')';

end

== matlab function px4_mc_notch_sim/PX4 Controllers/Linear Velocity Controller/MATLAB Function ==
  data: fx input; fx_sat output; fy input; fz input; fy_sat output; fz_sat output; MPC_THR_MAX parameter; MPC_THR_MIN parameter; MPC_TILTMAX_AIR parameter
function [fx_sat, fy_sat, fz_sat] = constrain_max_tilt(fx, fy, fz,MPC_THR_MAX, MPC_THR_MIN,MPC_TILTMAX_AIR)
    % First constrain fz.
    if fz > -MPC_THR_MIN
        fz_sat = -MPC_THR_MIN;
    elseif fz < -MPC_THR_MAX
        fz_sat = -MPC_THR_MAX;
    else
        fz_sat = fz;
    end
    
    % Constrain fx and fy
    thrust_max_NE_tilt = abs(fz_sat) * tan(MPC_TILTMAX_AIR * pi/180);
    thrust_max_NE = sqrt(MPC_THR_MAX*MPC_THR_MAX - fz_sat*fz_sat);
    thrust_max_NE = min(thrust_max_NE_tilt, thrust_max_NE);
    
    fx_sat = fx;
    fy_sat = fy;
    
    if dot([fx, fy], [fx, fy]) > thrust_max_NE*thrust_max_NE
        mag = norm([fx, fy]);
        fx_sat = fx / mag * thrust_max_NE;
        fy_sat = fy / mag * thrust_max_NE;
    end
end

== matlab function px4_mc_notch_sim/PX4 Controllers/Conversion: Thrust to Attitude/thrust2att ==
  data: force input size=3; quat output size=4; yaw input size=1; thrust output size=1
function [quat, thrust] = thrust2att(force, yaw)
    coder.extrinsic('dcm2quat');

% Read: Minimum  Snap  Trajectory  Generation  and  Control  for
% Quadrotors by Daniel Mellinger and Vijay Kumar to understand

        % Initialise quat
    quat = [1; 0; 0; 0];
    
    % Thrust is norm of force
    thrust = norm(force);
    
    % Determine body_z rotation (fit body_z onto z axis of force)
    if thrust > 1e-6
        body_z = -force./thrust;
    else
       body_z = [0; 0; 1]; 
    end
    
    % Determine body_x
    yaw_dir = [-sin(yaw); cos(yaw); 0];
    
    if abs(body_z(3)) > 1e-6
        body_x = cross(yaw_dir, body_z);
        
        if body_z(3) < 0
            body_x = -body_x;
        end
        body_x = body_x ./ norm(body_x);
    else
        body_x = [0; 0; 1];
    end
    
    % Determine body_y
    body_y = cross(body_z, body_x);
    body_y = body_y ./ norm(body_y);
    
    % Calculate rotation
    dcm = [body_x body_y body_z];
    quat = dcm2quat(dcm');
    
    % Normalise quaternion
    quat = quat ./ norm(quat);
    
end

== matlab function px4_mc_notch_sim/PX4 Controllers/Attitude Controller/Error Quaternion Calculation ==
  data: quat input; quat_sp input; quat_e output; thrust input; thrust_out output
function [quat_e, thrust_out] = error_quat(quat, quat_sp, thrust)
    if quat_sp == [0; 0; 0; 0]
       quat_sp = [1; 0; 0; 0];
    end
    
    quat_e = quatmultiply([quat(1) -quat(2) -quat(3) -quat(4)]./norm(quat), quat_sp');
    thrust_out = thrust;
end

== matlab function px4_mc_notch_sim/PX4 Controllers/Mixin Matrix/Mixin_mat ==
  data: dT input; thrust output; dA input; dE input; dR input; mixin_matrix parameter
function thrust = mixin_mat(dT, dA, dE, dR, mixin_matrix)

    thrust = mixin_matrix * [dT; dA; dE; dR];

end

== matlab function px4_mc_notch_sim/Disturbance Generator/MATLAB Function ==
  data: x input; forces output; z input; a input; b input; moments output
function [forces,moments] = fcn(x,z,a,b)
    % x : activate disturbance
    % y : activate disturbance rejection
    % z : disturbance type selector
    % a : disturbance moment selector
    % b : disturbance force selector
    if x
        % Moments
        if a == 1
            moments = [1;0;0];
        elseif a == 2
            moments = [0;1;0];
        elseif a == 3
            moments = [0;0;1];
        else 
            moments = [0;0;0];
        end
        
        % Forces
        if b == 5
            forces = [1;0;0];
        elseif b == 6
            forces = [0;1;0];
        elseif b == 7 
            forces = [0;0;1];
        else
            forces = [0;0;0];
        end
        
    else
        forces= [0;0;0];
        moments = [0;0;0];
    end
    
    forces = z*forces;
    moments = z*moments;
    
end
